simulink model "car_sus"  (Simulink 8.3)
settings: Solver=ode45  StartTime=0.0  StopTime=3  RelTol=1e-3
values from neighbouring files (symbols this model uses):
  A = [-1 1 0;-1 0 0;0 -1 -1]    [bookEx.m]    (also in carsus.m = [ 0 1 0 0; [-ks -bs ks bs]/mb ;        0 0 0 1; [ks bs -ks-k; massSpring.m = [0 0 1 0)
  B = [-1;0;0]    [bookEx.m]    (also in carsus.m = [0 0; 0 10000/mb ; 0 0; [kt -10000]/mw]; massSpring.m = [0;0;0;k/m])
  C = [1 0 0;0 0 1]    [bookEx.m]    (also in carsus.m = eye(4); massSpring.m = [1 0 0 0;0 1 0 0;0 0 1 0;0 0 0 1])
  E = B    [bookEx.m]    (also in carsus.m = [1;1;1;1]; massSpring.m = [0;0;0;1])
  F = A1-K1*C    [bookEx.m]    (also in carsus.m = diag(v); massSpring.m)
  H = E*inv((C*E)'*(C*E))*(C*E)'    [bookEx.m]    (also in carsus.m; massSpring.m)
  k = k1+k2    [carsus.m]    (also in massSpring.m = 1)
  K1 = place(A',C',[-2,-10,-5])'    [bookEx.m]    (also in massSpring.m = place(A',C',[-2,-10,-5,-3])')
  T = eye(3)-H*C    [bookEx.m]    (also in carsus.m = eye(4)-H*C; massSpring.m = eye(4)-H*C)
  X_0 = [-1;10;3;5]    [carsus.m]
settings Model: Creator=sqn4594  LastModifiedBy=sqn4594
settings OptimizationCC: InitFltsAndDblsToZero=on
settings DebuggingCC: SaveWithParameterizedLinksMsg=none  SignalResolutionControl=TryResolveAllWithWarning  MultiTaskDSMMsg=warning  MultiTaskCondExecSysMsg=none  StateNameClashWarn=none
settings RTWCC: IncludeERTFirstTime=on
settings GRTTargetCC: TargetFcnLib=ansi_tfl_tmw.mat

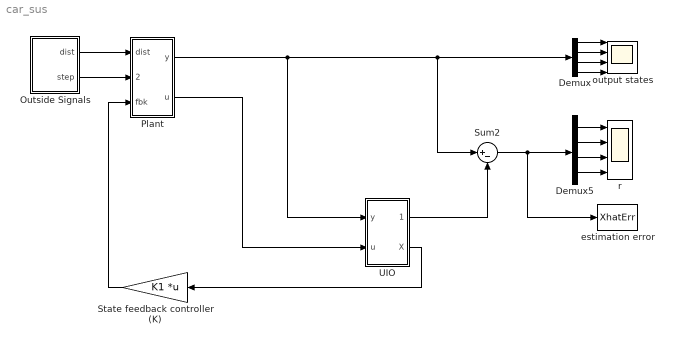
== system car_sus ==
  Demux : Demux
  Demux5 : Demux
  Outside Signals : Subsystem
  Plant : Subsystem
  State feedback controller (K) : Gain  Gain=K1  Multiplication=Matrix(K*u)
  Sum2 : Sum  Inputs=|+-
  UIO : Subsystem
  estimation error : ToWorkspace  VariableName=XhatErr  SampleTime=-1
  output states : Scope  NumInputPorts=4
      settings: TimeRange=10  YMin=-5~-5~-5~-5  YMax=5~5~5~5
  r : Scope  NumInputPorts=4
      settings: YMin=-5~-5~-5~-5  YMax=5~5~5~5  SaveName=ScopeData5
  wires:
  Plant/1(y) -> UIO/1(y), Demux/1, Sum2/1
  Demux/2 -> output states/2
  Demux/3 -> output states/3
  Demux/4 -> output states/4
  Plant/2(u) -> UIO/2(u)
  UIO/1(ydot) -> Sum2/2
  Demux5/1 -> r/1
  Demux5/2 -> r/2
  Demux5/3 -> r/3
  Demux5/4 -> r/4
  Sum2/1 -> Demux5/1, estimation error/1
  Demux/1 -> output states/1
  Outside Signals/2("step ") -> Plant/2(step)
  Outside Signals/1(dist) -> Plant/1(dist)
  UIO/2(X) -> State feedback controller (K)/1
  State feedback controller (K)/1 -> Plant/3(fbk)

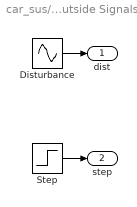
== system car_sus/Outside Signals ==
  Disturbance : Sin  Frequency=100  SampleTime=0
  Step : Step  Time=0  SampleTime=0
  dist : Outport
  "step " : Outport  Port=2
  wires:
  Disturbance/1 -> dist/1
  Step/1 -> "step "/1

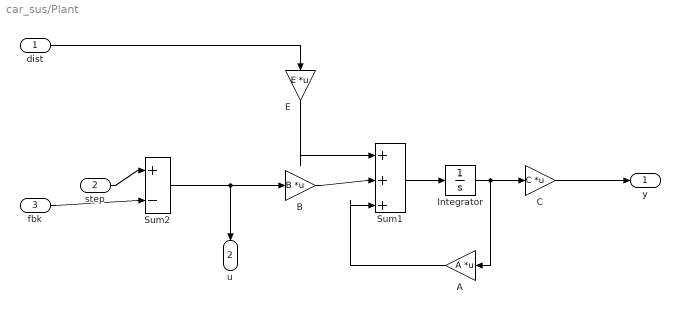
== system car_sus/Plant ==
  dist : Inport
  step : Inport  Port=2
  fbk : Inport  Port=3
  A : Gain  Gain=A  Multiplication=Matrix(K*u)
  B : Gain  Gain=B  Multiplication=Matrix(K*u)
  C : Gain  Gain=C  Multiplication=Matrix(K*u)
  E : Gain  Gain=E  Multiplication=Matrix(K*u)
  Integrator : Integrator  InitialCondition=X_0
  Sum1 : Sum  Inputs=|+++
  Sum2 : Sum  Inputs=|+-
  y : Outport
  u : Outport  Port=2
  wires:
  Sum1/1 -> Integrator/1
  step/1 -> Sum2/1
  fbk/1 -> Sum2/2
  Integrator/1 -> C/1, A/1
  B/1 -> Sum1/2
  Sum2/1 -> B/1, u/1
  A/1 -> Sum1/3
  E/1 -> Sum1/1
  C/1 -> y/1
  dist/1 -> E/1

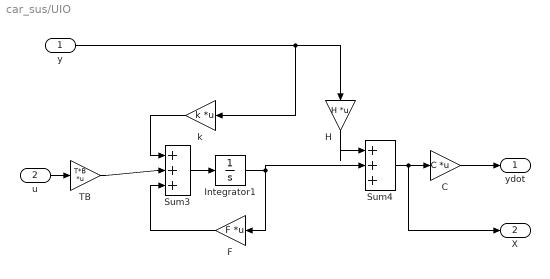
== system car_sus/UIO ==
  y : Inport
  u : Inport  Port=2
  C : Gain  Gain=C  Multiplication=Matrix(K*u)
  F : Gain  Gain=F  Multiplication=Matrix(K*u)
  H : Gain  Gain=H  Multiplication=Matrix(K*u)
  Integrator1 : Integrator
  Sum3 : Sum  Inputs=|+++
  Sum4 : Sum  Inputs=|+++
  TB : Gain  Gain=T*B  Multiplication=Matrix(K*u)
  k : Gain  Gain=k  Multiplication=Matrix(K*u)
  ydot : Outport
  X : Outport  Port=2
  wires:
  Sum3/1 -> Integrator1/1
  Integrator1/1 -> F/1, Sum4/2
  F/1 -> Sum3/3
  k/1 -> Sum3/1
  TB/1 -> Sum3/2
  H/1 -> Sum4/1
  Sum4/1 -> X/1, C/1
  y/1 -> H/1, k/1
  u/1 -> TB/1
  C/1 -> ydot/1
